simulink model "EnvelopeRecognition"  (Simulink 8.6)
settings: Solver=FixedStepDiscrete  StartTime=0.0  StopTime=10.0  RelTol=1e-3
undefined symbols (not defined in the file or in its folder): Rec, SDTV
libraries: visiontextngfix x3, visionconversions x3, visionsinks x2, visionmorphops x1, visionsources x1, dspmtrx3 x1
settings Model: Creator=Vitali  LastModifiedBy=Anton
settings DebuggingCC: SolverPrmCheckMsg=none  FcnCallInpInsideContextMsg=UseLocalSettings

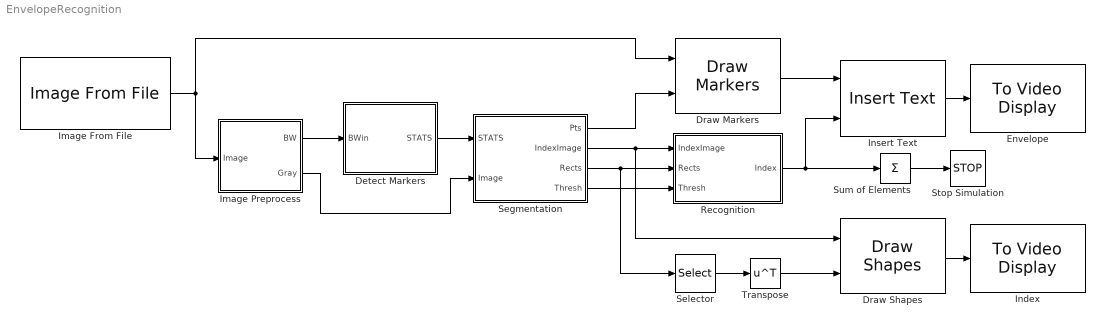
== system EnvelopeRecognition ==
  Detect Markers : Subsystem
  Draw Markers : visiontextngfix/Draw Markers  shape=Plus  size=3  fill=off  fillClrSource=Specify via dialog  display=White  intensity=200  color=[200 255 100]  opacity=0.6  viewport=Entire image  antialiasing=off  inType=Obsolete  imagePorts=One multidimensional signal  prodOutputMode=Binary point scaling  prodOutputWordLength=32  prodOutputFracLength=14  memoryMode=Specify word length  memoryWordLength=16  memoryFracLength=15  roundingMode=Floor  overflowMode=off
  Draw Shapes : visiontextngfix/Draw Shapes  shape=Rectangles  fill=off  lineWidth=1  fillClrSource=Specify via dialog  display=Black  intensity=200  color=[200 255 100]  opacity=0.6  viewport=Entire image  antialiasing=off  inType=Obsolete  imagePorts=One multidimensional signal  prodOutputMode=Binary point scaling  prodOutputWordLength=32  prodOutputFracLength=14  memoryMode=Specify word length  memoryWordLength=16  memoryFracLength=15  roundingMode=Floor  overflowMode=off
  Envelope : visionsinks/To Video Display  windowSizeMode=True size (1:1)  openAtMdlStart=on  fullScreen=off  videoWindowX=44  videoWindowY=90  saveWindowSize=off  videoWindowWidth=1152  videoWindowHeight=757  inputColorFormat=RGB  inputType=Obsolete  imagePorts=One multidimensional signal  OutputDevice=On-screen video monitor  dataOrg=Column-major  isWindowOpen=off
  Image From File : visionsources/Image From File  Tag=vipblks_nd  FileName=..\Images\DSC00390.JPG  imagePorts=One multidimensional signal  Ts=inf  ImageDataType=Inherit from input image  Signed=on  WordLength=16  sdImageDataType=uint(8)  FractionLengthMode=User-defined  FractionLength=15  OutPortLabels=R|G|B
  Image Preprocess : Subsystem
  Index : visionsinks/To Video Display  windowSizeMode=True size (1:1)  openAtMdlStart=on  fullScreen=off  videoWindowX=221  videoWindowY=385  saveWindowSize=off  videoWindowWidth=217  videoWindowHeight=65  inputColorFormat=RGB  inputType=Obsolete  imagePorts=One multidimensional signal  OutputDevice=On-screen video monitor  dataOrg=Column-major  isWindowOpen=off
  Insert Text : visiontextngfix/Insert Text  inputType=Obsolete  theText='%s'  getTextLocFrom=Specify via dialog  textLoc=[1 1]  getTextColorFrom=Specify via dialog  textColor=[0 255 0]  getTextIntensityFrom=Specify via dialog  textIntensity=0  getTextOpacityFrom=Specify via dialog  textOpacity=1.0  dummyVar2=0  dummyVar3=0  dummyVar4=0  imagePorts=One multidimensional signal  isInputTransposed=off  fontFace=LucidaSansRegular  dummyVar1=0  blockFontSize=24  antiAliased=on
  Recognition : Subsystem
  Segmentation : Subsystem
  Selector : Selector  NumberOfDimensions=2  InputPortWidth=3  IndexOptions=Index vector (dialog),Select all  Indices=[2, 1, 4, 3],  OutputSizes=1,1
  Stop Simulation : Stop
  Sum of Elements : Sum  Inputs=+  OutDataTypeStr=double
  Transpose : Math  Operator=transpose  SaturateOnIntegerOverflow=on
  wires:
  Image From File/1 -> Draw Markers/1, Image Preprocess/1(Image)
  Image Preprocess/1(BW) -> Detect Markers/1(BWin)
  Detect Markers/1(STATS) -> Segmentation/1(STATS)
  Segmentation/1(Pts) -> Draw Markers/2
  Image Preprocess/2(Gray) -> Segmentation/2(Image)
  Draw Shapes/1 -> Index/1
  Segmentation/2(IndexImage) -> Draw Shapes/1, Recognition/1(IndexImage)
  Segmentation/3(Rects) -> Selector/1, Recognition/2(Rects)
  Segmentation/4(Thresh) -> Recognition/3(Thresh)
  Draw Markers/1 -> Insert Text/1
  Insert Text/1 -> Envelope/1
  Recognition/1(Index) -> Insert Text/2, Sum of Elements/1
  Sum of Elements/1 -> Stop Simulation/1
  Selector/1 -> Transpose/1
  Transpose/1 -> Draw Shapes/2

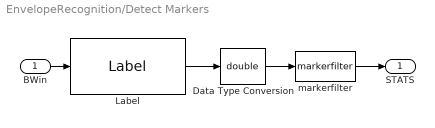
== system EnvelopeRecognition/Detect Markers ==
  BWin : Inport
  Data Type Conversion : DataTypeConversion  OutDataTypeStr=double
  Label : visionmorphops/Label  conn=8  output=Label matrix  outType=Automatic  lastLabel=maximum value of the output data type
  markerfilter : MATLABFcn  MATLABFcn=markerfilter  OutputDimensions=[7, 7]  Output1D=off
  STATS : Outport
  wires:
  BWin/1 -> Label/1
  Label/1 -> Data Type Conversion/1
  markerfilter/1 -> STATS/1
  Data Type Conversion/1 -> markerfilter/1

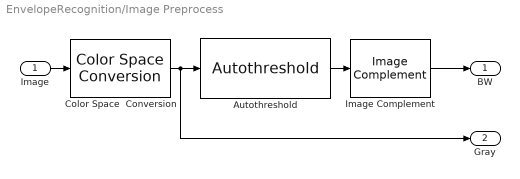
== system EnvelopeRecognition/Image Preprocess ==
  Image : Inport
  Autothreshold : visionconversions/Autothreshold  operator=>  threshOut=off  effMetricOut=off  userDefinedRange=off  umin=0  umax=255  outOfRngOpt=Warn and saturate  scaleThreshold=off  scaleFactor=1  P1Mode=Specify word length  P1WordLength=32  P1FracLength=30  P2Mode=Specify word length  P2WordLength=32  P2FracLength=22  P3Mode=Specify word length  P3WordLength=32  P3FracLength=14  P4Mode=Binary point scaling  P4WordLength=32  P4FracLength=15  Q1Mode=Specify word length  Q1WordLength=32  Q1FracLength=16  EMMode=Specify word length  EMWordLength=16  EMFracLength=14  roundingMode=Floor  overflowMode=off
  Color Space  Conversion : visionconversions/Color Space  Conversion  conversion=Obsolete  conversionActive=R'G'B' to intensity  wp_str=D65  rec=Rec. 601 (SDTV)  sys=1125/60/2:1  imagePorts=One multidimensional signal
  Image Complement : visionconversions/Image Complement
  BW : Outport
  Gray : Outport  Port=2
  wires:
  Image/1 -> Color Space  Conversion/1
  Color Space  Conversion/1 -> Autothreshold/1, Gray/1
  Autothreshold/1 -> Image Complement/1
  Image Complement/1 -> BW/1

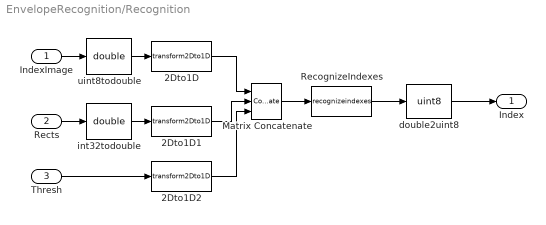
== system EnvelopeRecognition/Recognition ==
  IndexImage : Inport
  Rects : Inport  Port=2
  Thresh : Inport  Port=3
  2Dto1D : MATLABFcn  MATLABFcn=transform2Dto1D
  2Dto1D1 : MATLABFcn  MATLABFcn=transform2Dto1D
  2Dto1D2 : MATLABFcn  MATLABFcn=transform2Dto1D
  Matrix Concatenate : Concatenate  NumInputs=3  ConcatenateDimension=2
  RecognizeIndexes : MATLABFcn  MATLABFcn=recognizeindexes  OutputDimensions=[1, 6]  Output1D=off
  double2uint8 : DataTypeConversion  OutDataTypeStr=uint8
  int32todouble : DataTypeConversion  OutDataTypeStr=double
  uint8todouble : DataTypeConversion  OutDataTypeStr=double
  Index : Outport
  wires:
  IndexImage/1 -> uint8todouble/1
  Rects/1 -> int32todouble/1
  Thresh/1 -> 2Dto1D2/1
  2Dto1D1/1 -> Matrix Concatenate/2
  2Dto1D/1 -> Matrix Concatenate/1
  Matrix Concatenate/1 -> RecognizeIndexes/1
  RecognizeIndexes/1 -> double2uint8/1
  uint8todouble/1 -> 2Dto1D/1
  int32todouble/1 -> 2Dto1D1/1
  2Dto1D2/1 -> Matrix Concatenate/3
  double2uint8/1 -> Index/1

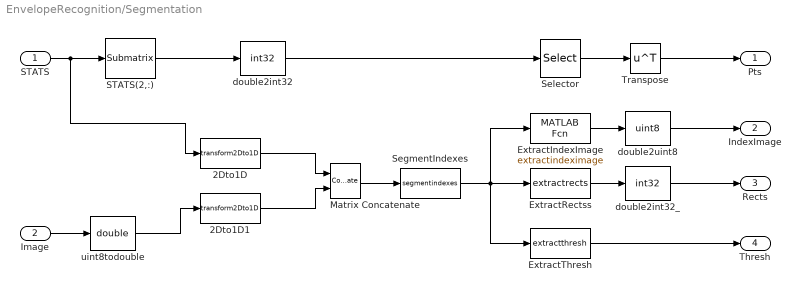
== system EnvelopeRecognition/Segmentation ==
  STATS : Inport
  Image : Inport  Port=2
  2Dto1D : MATLABFcn  MATLABFcn=transform2Dto1D
  2Dto1D1 : MATLABFcn  MATLABFcn=transform2Dto1D
  ExtractIndexImage : MATLABFcn  MATLABFcn=extractindeximage  OutputDimensions=[65 217]  Output1D=off
  ExtractRectss : MATLABFcn  MATLABFcn=extractrects  OutputDimensions=[4 7]  Output1D=off
  ExtractThresh : MATLABFcn  MATLABFcn=extractthresh  OutputDimensions=[1 1]  Output1D=off
  Matrix Concatenate : Concatenate  ConcatenateDimension=2
  STATS(2,:) : dspmtrx3/Submatrix  RowSpan=Range of rows  RowStartMode=First  RowStartIndex=1  RowEndMode=Index  RowEndIndex=2  ColSpan=All columns  ColStartMode=First  ColStartIndex=1  ColEndMode=Last  ColEndIndex=1
  SegmentIndexes : MATLABFcn  MATLABFcn=segmentindexes  OutputDimensions=[65*217+4*7+1, 1]  Output1D=off
  Selector : Selector  NumberOfDimensions=2  InputPortWidth=3  IndexOptions=Index vector (dialog),Select all  Indices=[2,1],1  OutputSizes=1,1
  Transpose : Math  Operator=transpose  SaturateOnIntegerOverflow=on
  double2int32 : DataTypeConversion  OutDataTypeStr=int32
  double2int32_ : DataTypeConversion  OutDataTypeStr=int32
  double2uint8 : DataTypeConversion  OutDataTypeStr=uint8
  uint8todouble : DataTypeConversion  OutDataTypeStr=double
  Pts : Outport
  IndexImage : Outport  Port=2
  Rects : Outport  Port=3
  Thresh : Outport  Port=4
  wires:
  STATS/1 -> STATS(2,:)/1, 2Dto1D/1
  STATS(2,:)/1 -> double2int32/1
  Image/1 -> uint8todouble/1
  2Dto1D/1 -> Matrix Concatenate/1
  2Dto1D1/1 -> Matrix Concatenate/2
  Matrix Concatenate/1 -> SegmentIndexes/1
  uint8todouble/1 -> 2Dto1D1/1
  SegmentIndexes/1 -> ExtractIndexImage/1, ExtractRectss/1, ExtractThresh/1
  ExtractIndexImage/1 -> double2uint8/1
  ExtractThresh/1 -> Thresh/1
  ExtractRectss/1 -> double2int32_/1
  double2uint8/1 -> IndexImage/1
  double2int32/1 -> Selector/1
  Selector/1 -> Transpose/1
  double2int32_/1 -> Rects/1
  Transpose/1 -> Pts/1
